simulink model "chap16_3sim"  (Simulink 7.7)
settings: Solver=ode113  StartTime=0.0  StopTime=30  RelTol=1e-5
settings Model: Creator=hp  LastModifiedBy=ljk  ExtModeTrigMode=oneshot  ExtModeArmWhenConnect=off
settings DataIOCC: LimitDataPoints=off  SignalLoggingName=sigsOut
settings OptimizationCC: BooleanDataType=off  InitFltsAndDblsToZero=on
settings DebuggingCC: SaveWithParameterizedLinksMsg=none  SignalResolutionControl=TryResolveAllWithWarning  SolverPrmCheckMsg=none  MultiTaskDSMMsg=warning  MultiTaskCondExecSysMsg=none  StrictBusMsg=Warning
settings HardwareCC: TargetUnknown=on
settings RTWCC: IncludeERTFirstTime=on
settings GRTTargetCC: TargetFcnLib=ansi_tfl_tmw.mat

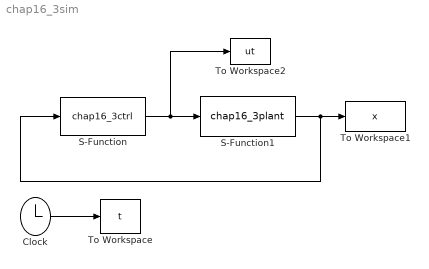
== system chap16_3sim ==
  Clock : Clock
      settings: Decimation=30
  S-Function : S-Function  FunctionName=chap16_3ctrl  EnableBusSupport=off
  S-Function1 : S-Function  FunctionName=chap16_3plant  EnableBusSupport=off
  To Workspace : ToWorkspace  VariableName=t  SampleTime=-1  SaveFormat=Array
  To Workspace1 : ToWorkspace  VariableName=x  SampleTime=-1  SaveFormat=Array
  To Workspace2 : ToWorkspace  VariableName=ut  SampleTime=-1  SaveFormat=Array
  wires:
  S-Function/1 -> S-Function1/1, To Workspace2/1
  S-Function1/1 -> S-Function/1, To Workspace1/1
  Clock/1 -> To Workspace/1
